simulink model "OneRobot_feedback"  (R2014b)
settings: Solver=ode45  StartTime=0.2  StopTime=10  FixedStep=0.01  RelTol=1e-3
settings Model: Creator=mshahria  LastModifiedBy=mshahria

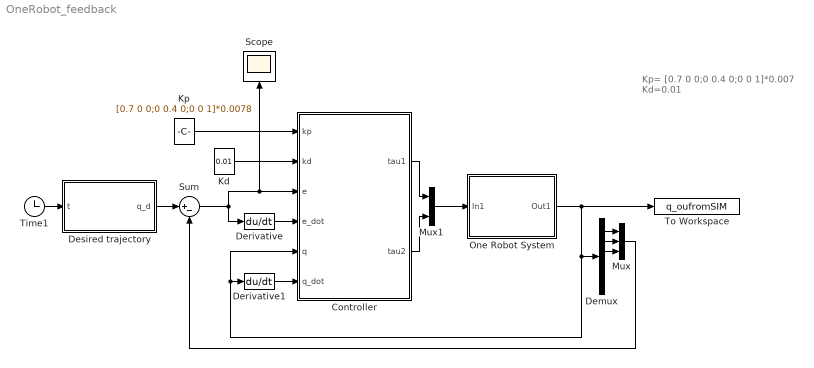
== system OneRobot_feedback ==
  note: Kp= [0.7 0 0;0 0.4 0;0 0 1]*0.007
      | Kd=0.01
  " One Robot System" : Subsystem
  "Controller " : MATLAB Function  TreatAsAtomicUnit=on
  Demux : Demux  Outputs=6
  Derivative : Derivative
  Derivative1 : Derivative
  Desired trajectory : MATLAB Function  TreatAsAtomicUnit=on
  Kd : Constant  Value=0.01
  Kp : Constant  Value=[0.7 0 0;0 0.4 0;0 0 1]*0.0078
  Mux : Mux  Inputs=3
  Mux1 : Mux  Inputs=2
  Scope : Scope
  Sum : Sum  Inputs=|+-
  Time1 : Clock
  To Workspace : ToWorkspace  VariableName=q_oufromSIM  SampleTime=-1
  wires:
  " One Robot System"/1(Out1) -> To Workspace/1, Demux/1, Derivative1/1, "Controller "/5(q)
  Time1/1 -> Desired trajectory/1(t)
  Demux/1 -> Mux/1
  Demux/2 -> Mux/2
  Mux/1 -> Sum/2
  Demux/3 -> Mux/3
  Desired trajectory/1(q_d) -> Sum/1
  Sum/1 -> "Controller "/3(e), Scope/1, Derivative/1
  Kd/1 -> "Controller "/2(kd)
  Derivative/1 -> "Controller "/4(e_dot)
  Derivative1/1 -> "Controller "/6(q_dot)
  "Controller "/1(tau1) -> Mux1/1
  "Controller "/2(tau2) -> Mux1/2
  Mux1/1 -> " One Robot System"/1(In1)
  Kp/1 -> "Controller "/1(kp)

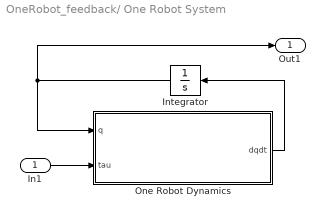
== system OneRobot_feedback/ One Robot System ==
  In1 : Inport
  Integrator : Integrator  InitialCondition=|  LimitOutput=on  UpperSaturationLimit=[inf,inf,inf,0.4,0.4,0.5]  LowerSaturationLimit=[-inf,-inf,-inf,-0.4,-0.4,-0.5]
      | [.2136; 0.7015
      | ;pi/3;0;0;0]
  One Robot Dynamics : MATLAB Function  TreatAsAtomicUnit=on
  Out1 : Outport
  wires:
  Integrator/1 -> Out1/1, One Robot Dynamics/1(q)
  One Robot Dynamics/1(dqdt) -> Integrator/1
  In1/1 -> One Robot Dynamics/2(tau)

== matlab function OneRobot_feedback/Desired trajectory ==
  data: t input; q_d output
function q_d = fcn(t)

q_d = q_desired(t);

== matlab function OneRobot_feedback/ One Robot System/One Robot Dynamics ==
  data: dqdt output; q input; tau input
function dqdt= Robot_ode(q,tau)
dqdt=zeros(6,1);
% global tau_l tau_r; 
tau_l=tau(1);
tau_r=tau(2);

x_dot=q(4);
y_dot=q(5);
theta=q(3);
theta_dot=q(6);
q_dotdot = Qdotdot(tau_l,tau_r,theta,theta_dot,x_dot,y_dot);

dqdt(1)=q(4);
dqdt(2)=q(5);
dqdt(3)=q(6);
dqdt(4)=(q_dotdot(1));
dqdt(5)=(q_dotdot(2));
dqdt(6)=(q_dotdot(3));

== matlab function OneRobot_feedback/Controller  ==
  data: kp input; kd input; e input; e_dot input; tau1 output; q input; q_dot input; tau2 output
function [tau1,tau2]= controller(kp,kd,e,e_dot,q,q_dot)

theta=q(3);
theta_dot=q(6);
x_dotdot=q_dot(4);
y_dotdot=q_dot(5);
theta_dotdot=q_dot(6);
x_dot=q(4);
y_dot=q(5);


B_inv=B_inverse(theta);
tau_compued = Tau_compued(theta,theta_dot,theta_dotdot,x_dot,x_dotdot,y_dot,y_dotdot) +B_inv*(kp*e+kd*e_dot) ;

tau1=tau_compued(1);
tau2=tau_compued(2);
